simulink library "libGravityModel"  (R2020b)
settings: Solver=VariableStepAuto  StartTime=0.0  StopTime=10.0  RelTol=1e-3
libraries: vrlib x2, aerolibconvert2 x1, aerolibtransform2 x1
settings Model: Creator=caatay  LastModifiedBy=caatay

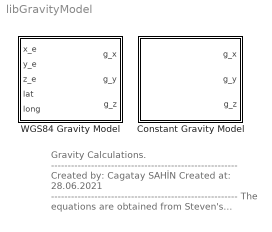
== system libGravityModel ==
  note: Gravity Calculations.
      | --------------------------------------------------------
      | Created by: Cagatay SAHİN
      | Created at: 28.06.2021
      | --------------------------------------------------------
      | The equations are obtained from
      | Steven's textbook.
      | The reference book can be found in
      | "references folder".
      | --------------------------------------------------------
      | for question:
      | cagataysahin44@gmail.com
  Constant Gravity Model : Subsystem  mask(Environment Model - Constant Gravity Model){g_x=0, g_y=0, g_z=32.17}
      mask prompts: g_x "Gravitional Acceleration on X-Axis"; g_y "Gravitional Acceleration on Y-Axis"; g_z "Gravitional Acceleration on Z-Axis"
      mask help: Low-fidelity gravity model which has only constant gravity value on z-axis.
      mask Help:
      | This block use constant value to obtain gravitional accelearion on z-axis.
      | --------------------------------------------------------------------------------------------------------------------------------------------------
      | Output of the function:
      | 	g_x: Gravity on X-Axis (ft/s^2)
      |                   g_y: Gravity on Y-Axis (ft/s^2)
      | 	g_z: Gravity on Z-Axis (ft/s^2)
      | --------------------------------------------------------------------------------------------------------------------------------------------------
      | All equations can be found in Steven's text book. Reference can be found in "literature" subfolder.
      | for question: "cagataysahin44@gmail.com"
      mask DialogControl Container2 Prompt: Parameters
      mask Display:
      | port_label('output',1,'g_{x}','texmode','on');
      | port_label('output',2,'g_{y}','texmode','on');
      | port_label('output',3,'g_{z}','texmode','on');
  WGS84 Gravity Model : Subsystem  mask(Environment Model - WGS84 Gravity Model){h_0=0, a=6378137, b=6356752, w_e=[0; 0; 7.29115e-05], GM=3986004.418e8, R_e=6378137, J_2=1.082626684e-3}
      mask prompts: h_0 "Initial Estimation Altitude (ft)"; a "Semi-Major Axis (m)"; b "Semi-Minor Axis (m)"; w_e "Earth's Angular Rate (rad/s)"; GM "Gravitional Constant (m^3/s^2)"; R_e "Radius of Earth (m)"; J_2 "J2 Constant"
      mask help: High Fidelity Gravity Model which is referenced by WGS84 Gravity Model. The model are obtained with using NED position and latitude and longitude information.
      mask Help:
      | This block is used for obtain high fidelity gravity parameters with using state information.
      | --------------------------------------------------------------------------------------------------------------------------------------------------
      | Input of the function:
      | 	x_e: North Position (ft)
      | 	y_e: East Position (ft)
      | 	z_e: Down Position (ft)
      | 	lat:Latitude (rad)
      | 	long: Longitude (rad)
      | Outputs => Gravity on X-Axis (ft/s^2)
      |                     Gravity on Y-Axis (ft/s^2)
      | 	  Gravity on Z-Axis (ft/s^2)
      | --------------------------------------------------------------------------------------------------------------------------------------------------
      | All equations can be found in Steven's text book. Reference can be found in "literature" subfolder.
      | for question: "cagataysahin44@gmail.com"
      mask DialogControl Container2 Prompt: Parameters
      mask Display:
      | port_label('input',1,'x_{e}','texmode','on');
      | port_label('input',2,'y_{e}','texmode','on');
      | port_label('input',3,'z_{e}','texmode','on');
      | port_label('input',4,'\mu','texmode','on');
      | port_label('input',5,'l','texmode','on');
      | 
      | port_label('output',1,'g_{x}','texmode','on');
      | port_label('output',2,'g_{y}','texmode','on');
      | port_label('output',3,'g_{z}','texmode','on');

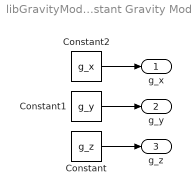
== system libGravityModel/Constant Gravity Model ==
  Constant : Constant  Value=g_z
  Constant1 : Constant  Value=g_y
  Constant2 : Constant  Value=g_x
  g_x : Outport  VectorParamsAs1DForOutWhenUnconnected=off
  g_y : Outport  Port=2  VectorParamsAs1DForOutWhenUnconnected=off
  g_z : Outport  Port=3  VectorParamsAs1DForOutWhenUnconnected=off
  wires:
  Constant/1 -> g_z/1
  Constant2/1 -> g_x/1
  Constant1/1 -> g_y/1

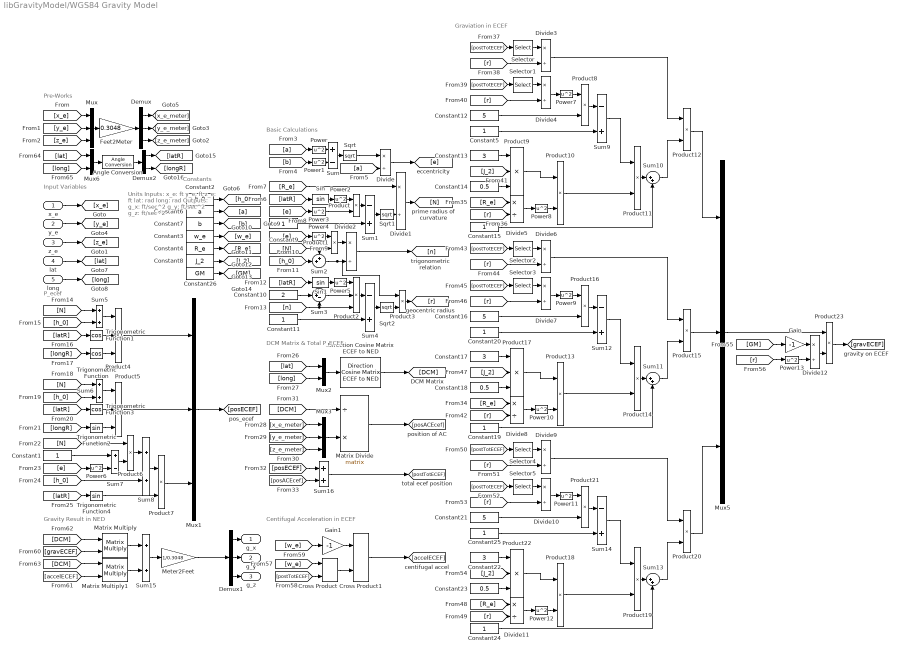
== system libGravityModel/WGS84 Gravity Model ==
  note: Gravity Result in NED
  note: Constants
  note: Graviation in ECEF
  note: Centifugal Acceleration in ECEF
  note: Pre-Works
  note: Input Variables
  note: DCM Matrix & Total P_ECEF
  note: Units
      | Inputs:
      | x_e: ft
      | y_e: ft
      | z_e: ft
      | lat: rad
      | long: rad
      | Outputs:
      | g_x: ft/sec^2
      | g_y: ft/sec^2
      | g_z: ft/sec^2
  note: Basic Calculations
  note: P_ecef
  "x_e " : Inport
  y_e : Inport  Port=2
  z_e : Inport  Port=3
  lat : Inport  Port=4
  long : Inport  Port=5
  Angle Conversion : aerolibconvert2/Angle Conversion  IU=deg  OU=rad
  Constant{1,5,9,11,15,19..20,24..25} (9 alike) : Constant
  Constant10 : Constant  Value=2
  Constant12 : Constant  Value=5
  Constant13 : Constant  Value=3
  Constant14 : Constant  Value=0.5
  Constant16 : Constant  Value=5
  Constant17 : Constant  Value=3
  Constant18 : Constant  Value=0.5
  Constant2 : Constant  Value=h_0
  Constant21 : Constant  Value=5
  Constant22 : Constant  Value=3
  Constant23 : Constant  Value=0.5
  Constant26 : Constant  Value=GM
  Constant3 : Constant  Value=w_e
  Constant4 : Constant  Value=R_e
  Constant6 : Constant  Value=a
  Constant7 : Constant  Value=b
  Constant8 : Constant  Value=J_2
  Cross Product : vrlib/Utilities/Cross Product
  Cross Product1 : vrlib/Utilities/Cross Product
  Demux : Demux  Outputs=3
  Demux1 : Demux  Outputs=3
  Demux2 : Demux  Outputs=2
  Direction Cosine Matrix ECEF to NED : aerolibtransform2/Direction Cosine Matrix ECEF to NED
      settings: SourceProductBaseCode=AE
  Divide{,1..12} (13 alike) : Product  Inputs=*/
  Feet2Meter : Gain  Gain=0.3048
  Gain : Gain  Gain=-1
  Gain1 : Gain  Gain=-1
  Matrix Divide : Product  Inputs=/*  Multiplication=Matrix(*)
  Matrix Multiply : Product  Multiplication=Matrix(*)
  Matrix Multiply1 : Product  Multiplication=Matrix(*)
  Meter2Feet : Gain  Gain=1/0.3048
  Mux{,1,3,5} (4 alike) : Mux  Inputs=3
  Mux2 : Mux  Inputs=2
  Mux6 : Mux  Inputs=2
  Power{,1..13} (14 alike) : Math  Operator=square  SaturateOnIntegerOverflow=on
  Product{,1,3,6..8,10..16,18..21,23} (18 alike) : Product
  Product{2,4..5,9,17,22} (6 alike) : Product  Inputs=3
  Selector : Selector  InputPortWidth=3  IndexOptions=Index vector (dialog)  Indices=[1]  OutputSizes=1
  Selector{1,3..5} (4 alike) : Selector  InputPortWidth=3  IndexOptions=Index vector (dialog)  Indices=[3]  OutputSizes=1
  Selector2 : Selector  InputPortWidth=3  IndexOptions=Index vector (dialog)  Indices=[2]  OutputSizes=1
  Sin : Trigonometry
  Sin1 : Trigonometry
  Sqrt : Sqrt  SaturateOnIntegerOverflow=on
  Sqrt1 : Sqrt  SaturateOnIntegerOverflow=on
  Sqrt2 : Sqrt  SaturateOnIntegerOverflow=on
  Sum : Sum  Inputs=+-
  Sum{1,4,9,12,14} (5 alike) : Sum  Inputs=-+
  Sum10 : Sum  Inputs=|++
  Sum11 : Sum  Inputs=|++
  Sum13 : Sum  Inputs=|++
  Sum{5..6,8,15..16} (5 alike) : Sum
  Sum2 : Sum  Inputs=++|
  Sum3 : Sum  Inputs=|+-
  Sum7 : Sum  Inputs=+-
  Trigonometric Function : Trigonometry  Operator=cos
  Trigonometric Function1 : Trigonometry  Operator=cos
  Trigonometric Function2 : Trigonometry
  Trigonometric Function3 : Trigonometry  Operator=cos
  Trigonometric Function4 : Trigonometry
  g_x : Outport  VectorParamsAs1DForOutWhenUnconnected=off
  g_y : Outport  Port=2  VectorParamsAs1DForOutWhenUnconnected=off
  g_z : Outport  Port=3  VectorParamsAs1DForOutWhenUnconnected=off
  wires:
  Demux2/2 -> [longR]
  [long] -> Mux6/2
  [accelECEF] -> Matrix Multiply1/2
  Matrix Multiply1/1 -> Sum15/2
  Mux6/1 -> Angle Conversion/1
  Direction Cosine Matrix ECEF to NED/1 -> [DCM]
  [gravECEF] -> Matrix Multiply/2
  [DCM] -> Matrix Multiply/1
  Mux2/1 -> Direction Cosine Matrix ECEF to NED/1
  [posECEF] -> Sum16/1
  Angle Conversion/1 -> Demux2/1
  Demux1/3 -> g_z/1
  Demux2/1 -> [latR]
  [x_e] -> Mux/1
  Constant8/1 -> [J_2]
  [z_e] -> Mux/3
  Demux1/1 -> g_x/1
  Power3/1 -> Product/2
  Constant9/1 -> Sum1/2
  [e] -> Power3/1
  [a] -> Divide/2
  Sqrt/1 -> Divide/1
  Sum/1 -> Sqrt/1
  Power/1 -> Sum/1
  Power1/1 -> Sum/2
  Constant4/1 -> [R_e]
  [b] -> Power1/1
  Constant6/1 -> [a]
  [a] -> Power/1
  Sum7/1 -> Product6/2
  [h_0] -> Sum8/2
  Divide2/1 -> [n]
  [longR] -> Trigonometric Function2/1
  Sum6/1 -> Product5/1
  Trigonometric Function2/1 -> Product5/3
  [N] -> Sum6/1
  Trigonometric Function3/1 -> Product5/2
  Sum5/1 -> Product4/1
  [longR] -> Trigonometric Function/1
  [h_0] -> Sum5/2
  Sum4/1 -> Sqrt2/1
  Mux1/1 -> [posECEF]
  lat/1 -> [lat]
  Power5/1 -> Product2/1
  Demux/2 -> [y_e_meter]
  Gain1/1 -> Cross Product1/1
  Constant10/1 -> Sum3/1
  Product2/1 -> Sum4/1
  Sum3/1 -> Product2/2
  Product1/1 -> Divide2/1
  Sum2/1 -> Product3/1, Divide2/2
  Divide9/1 -> Product20/1
  [N] -> Sum2/1, Product1/2
  [h_0] -> Sum2/2
  Divide1/1 -> [N]
  [R_e] -> Divide1/1
  Gain/1 -> Divide12/1
  [J_2] -> Product22/2
  [e] -> Power6/1
  Divide5/1 -> Power8/1
  [r] -> Divide7/2
  Product22/1 -> Product18/1
  Divide11/1 -> Power12/1
  Sum8/1 -> Product7/1
  Product10/1 -> Product11/2
  Constant16/1 -> Product16/2
  Constant18/1 -> Product17/3
  Sum15/1 -> Meter2Feet/1
  Sqrt1/1 -> Divide1/2
  [r] -> Divide11/2
  Power13/1 -> Divide12/2
  Trigonometric Function4/1 -> Product7/2
  Divide7/1 -> Power9/1
  Selector4/1 -> Divide9/1
  [w_e] -> Cross Product/1
  [latR] -> Trigonometric Function3/1
  Cross Product1/1 -> [accelECEF]
  Sum12/1 -> Product14/1
  [J_2] -> Product9/2
  [e] -> Power4/1
  [postTotECEF] -> Cross Product/2
  Product9/1 -> Product10/1
  [GM] -> Gain/1
  Constant23/1 -> Product22/3
  [r] -> Power13/1
  Product8/1 -> Sum9/1
  Power2/1 -> Product/1
  [r] -> Divide10/2
  Demux/3 -> [z_e_meter]
  Product23/1 -> [gravECEF]
  Sum10/1 -> Product12/2
  Divide12/1 -> Product23/2
  Constant21/1 -> Product21/2
  Constant26/1 -> [GM]
  Constant24/1 -> Sum13/2
  Constant14/1 -> Product9/3
  [postTotECEF] -> Selector3/1
  Power4/1 -> Product1/1
  Selector2/1 -> Divide6/1
  Product7/1 -> Mux1/3
  [r] -> Divide3/2
  [postTotECEF] -> Selector4/1
  Mux5/1 -> Product23/1
  Power11/1 -> Product21/1
  Trigonometric Function1/1 -> Product4/2
  Product12/1 -> Mux5/1
  Product20/1 -> Mux5/3
  Selector/1 -> Divide3/1
  Sum14/1 -> Product19/1
  Sum16/1 -> [postTotECEF]
  [latR] -> Trigonometric Function1/1
  y_e/1 -> [y_e]
  Demux1/2 -> g_y/1
  Sum13/1 -> Product20/2
  Product13/1 -> Product14/2
  Mux/1 -> Feet2Meter/1
  Product21/1 -> Sum14/1
  Matrix Divide/1 -> [posACEcef]
  [r] -> Divide9/2
  [r] -> Divide6/2
  [J_2] -> Product17/2
  Constant7/1 -> [b]
  Constant22/1 -> Product22/1
  Product3/1 -> [r]
  Constant2/1 -> [h_0]
  Product19/1 -> Sum13/1
  Feet2Meter/1 -> Demux/1
  Constant15/1 -> Sum10/2
  Product18/1 -> Product19/2
  Divide10/1 -> Power11/1
  Power12/1 -> Product18/2
  Trigonometric Function/1 -> Product4/3
  Product4/1 -> Mux1/1
  [postTotECEF] -> Selector5/1
  Selector5/1 -> Divide10/1
  [postTotECEF] -> Selector2/1
  Product16/1 -> Sum12/1
  [latR] -> Sin/1
  Constant20/1 -> Sum12/2
  Sin1/1 -> Power5/1
  Constant19/1 -> Sum11/2
  Divide/1 -> [e]
  Selector1/1 -> Divide4/1
  Product5/1 -> Mux1/2
  Product17/1 -> Product13/1
  Power9/1 -> Product16/1
  Sum1/1 -> Sqrt1/1
  z_e/1 -> [z_e]
  Sum9/1 -> Product11/1
  Product11/1 -> Sum10/1
  Product15/1 -> Mux5/2
  Product6/1 -> Sum8/1
  [r] -> Divide5/2
  Constant12/1 -> Product8/2
  Constant13/1 -> Product9/1
  [z_e_meter] -> Mux3/3
  [latR] -> Sin1/1
  [R_e] -> Divide5/1
  Power7/1 -> Product8/1
  Divide4/1 -> Power7/1
  "x_e "/1 -> [x_e]
  Constant3/1 -> [w_e]
  Product14/1 -> Sum11/1
  Constant1/1 -> Sum7/1
  Divide3/1 -> Product12/1
  [n] -> Sum3/2, Product2/3
  Constant25/1 -> Sum14/2
  [lat] -> Mux2/1
  Divide6/1 -> Product15/1
  Power10/1 -> Product13/2
  [R_e] -> Divide11/1
  [h_0] -> Sum6/2
  [long] -> Mux2/2
  [postTotECEF] -> Selector/1
  [x_e_meter] -> Mux3/1
  Constant17/1 -> Product17/1
  [w_e] -> Gain1/1
  Demux/1 -> [x_e_meter]
  [R_e] -> Divide8/1
  [y_e] -> Mux/2
  Sqrt2/1 -> Product3/2
  [y_e_meter] -> Mux3/2
  [DCM] -> Matrix Divide/1
  [N] -> Product6/1
  Matrix Multiply/1 -> Sum15/1
  [N] -> Sum5/1
  Divide8/1 -> Power10/1
  [r] -> Divide4/2
  Sin/1 -> Power2/1
  Meter2Feet/1 -> Demux1/1
  Sum11/1 -> Product15/2
  Constant5/1 -> Sum9/2
  Power6/1 -> Sum7/2
  long/1 -> [long]
  [r] -> Divide8/2
  [latR] -> Trigonometric Function4/1
  Selector3/1 -> Divide7/1
  Cross Product/1 -> Cross Product1/2
  Mux3/1 -> Matrix Divide/2
  [postTotECEF] -> Selector1/1
  [lat] -> Mux6/1
  [DCM] -> Matrix Multiply1/1
  [posACEcef] -> Sum16/2
  Power8/1 -> Product10/2
  Constant11/1 -> Sum4/2
  Product/1 -> Sum1/1
